simulink model "PID"  (R2023a)
settings: Solver=VariableStepAuto  StartTime=0.0  StopTime=10.0  RelTol=1e-3
settings Model: Creator=ag027  LastModifiedBy=ag027

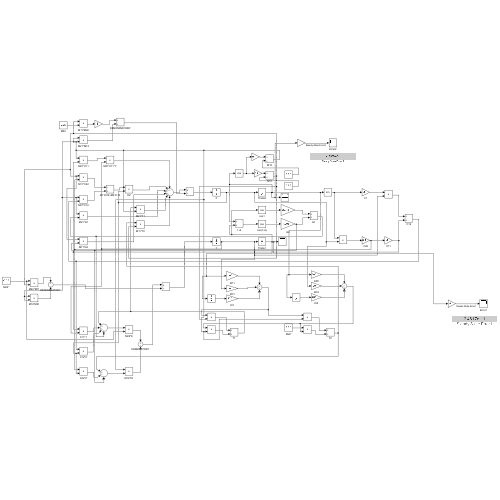
[thumbnail: Simulink's stored preview of the top-level diagram]
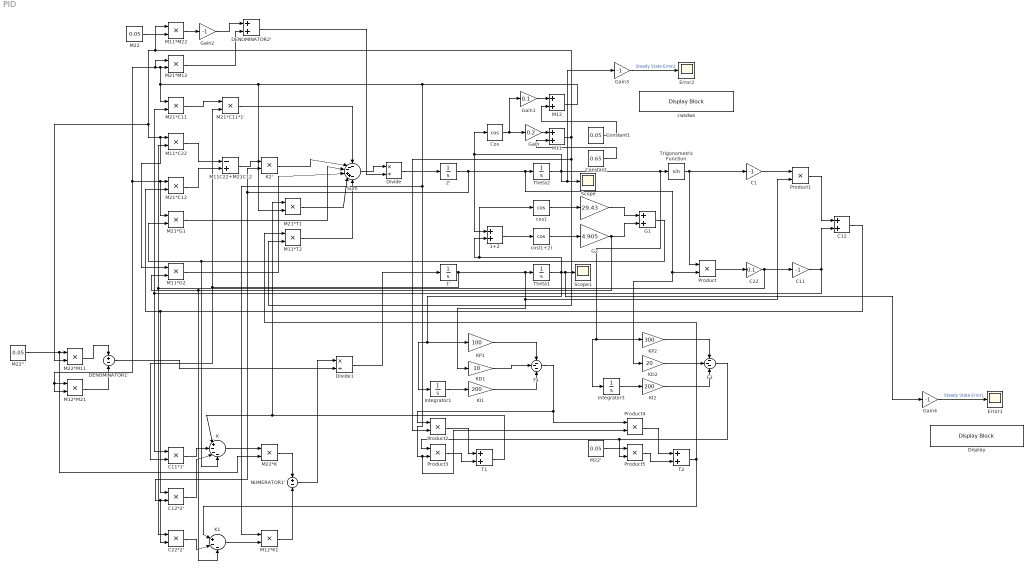
== system PID ==
  " " : Gain  Gain=29.43
  1' : Integrator
  1+2 : Sum
  2' : Integrator
  C1 : Gain  Gain=-1
  C11 : Gain  Gain=-1
  C11*1' : Product
  C12 : Sum
  C12*2' : Product
  C22 : Gain  Gain=0.1
  C22*2' : Product
  Constant : Constant  Value=0.65
  Constant1 : Constant  Value=0.05
  Cos : Trigonometry  Operator=cos
  DENOMINATOR1' : Sum  Inputs=+-
  DENOMINATOR2' : Sum
  Display : DisplayBlock  LabelPosition=Bottom  Transparency=1
  Divide : Product  Inputs=*/
  Divide1 : Product  Inputs=*/
  Error1 : Scope
  Error2 : Scope
  F1 : Sum  Inputs=---
  F2 : Sum  Inputs=---
  G1 : Sum
  G2 : Gain  Gain=4.905
  Gain : Gain  Gain=0.2
  Gain1 : Gain  Gain=0.1
  Gain2 : Gain  Gain=-1
  Gain3 : Gain  Gain=-1
  Gain4 : Gain  Gain=-1
  Integrator1 : Integrator
  Integrator3 : Integrator
  K : Sum  Inputs=|+---
  K1 : Sum  Inputs=|+--
  K2' : Product
  KD1 : Gain  Gain=10
  KD2 : Gain  Gain=20
  KI1 : Gain  Gain=200
  KI2 : Gain  Gain=200
  KP1 : Gain  Gain=100
  KP2 : Gain  Gain=300
  M11 : Sum
  M11*C22 : Product
  M11*G2 : Product
  M11*M22 : Product
  M11*T2 : Product
  M11C22+M21C12 : Sum  Inputs=-+
  M12 : Sum
  M12*K1 : Product
  M12*M21 : Product
  M21*C11 : Product
  M21*C11*1' : Product
  M21*C12 : Product
  M21*G1 : Product
  M21*M12 : Product
  M21*T1 : Product
  M22 : Constant  Value=0.05
  M22' : Constant  Value=0.05
  M22'' : Constant  Value=0.05
  M22*K : Product
  M22*M11 : Product
  NUMERATOR1' : Sum  Inputs=+-
  Product{,1..5} (6 alike) : Product
  Scope : Scope
  Scope1 : Scope
  Sum : Sum  Inputs=---++-
  T1 : Sum
  T2 : Sum
  Theta1 : Integrator  InitialCondition=0.1
  Theta2 : Integrator  InitialCondition=0.1
  Trigonometric Function : Trigonometry
  cos(1+2) : Trigonometry  Operator=cos
  cos1 : Trigonometry  Operator=cos
  cwsdws : DisplayBlock  LabelPosition=Bottom  Transparency=1
  wires:
  Constant/1 -> M11/2
  Cos/1 -> Gain1/1, Gain/1
  Gain/1 -> M11/1
  Gain1/1 -> M12/1
  Constant1/1 -> M12/2
  1'/1 -> Product1/2, KD1/1, Theta1/1, C11*1'/2, M21*C11*1'/2
  Theta1/1 -> Gain4/1, Scope1/1, cos1/1, 1+2/2, KP1/1, Integrator1/1
  1+2/1 -> cos(1+2)/1
  cos(1+2)/1 -> G2/1
  cos1/1 -> " "/1
  G2/1 -> M11*G2/2, K1/3, G1/2
  " "/1 -> G1/1
  Trigonometric Function/1 -> C1/1, Product/1
  Product/1 -> C22/1
  C22/1 -> C22*2'/1, M11*C22/2, C11/1
  C1/1 -> Product1/1
  Product1/1 -> C12/1
  C11/1 -> C12/2, C11*1'/1, M21*C11/2
  M12/1 -> Product4/2, Product3/2, M12*K1/1, M21*T1/2, M21*C11/1, M12*M21/2, M12*M21/1, M21*G1/1, M21*C12/1, M21*M12/1, M21*M12/2
  M11/1 -> M11*T2/2, Product2/2, M22*M11/2, M11*G2/1, M11*C22/1, M11*M22/1
  M22/1 -> M11*M22/2
  M11*M22/1 -> Gain2/1
  Gain2/1 -> DENOMINATOR2'/1
  M21*M12/1 -> DENOMINATOR2'/2
  M21*C11/1 -> M21*C11*1'/1
  M21*C11*1'/1 -> Sum/1
  C12/1 -> C12*2'/1, M21*C12/2
  M11*C22/1 -> M11C22+M21C12/1
  M21*C12/1 -> M11C22+M21C12/2
  M11C22+M21C12/1 -> K2'/1
  K2'/1 -> Sum/2
  G1/1 -> K/4, M21*G1/2
  M21*G1/1 -> Sum/3
  M11*G2/1 -> Sum/4
  Integrator1/1 -> KI1/1
  KP1/1 -> F1/1
  KD1/1 -> F1/2
  KI1/1 -> F1/3
  KI2/1 -> F2/3
  Integrator3/1 -> KI2/1
  2'/1 -> C22*2'/2, C12*2'/2, K2'/2, Product/2, KD2/1, Theta2/1
  KP2/1 -> F2/1
  KD2/1 -> F2/2
  F1/1 -> Product4/1, Product2/1
  F2/1 -> Product5/2, Product3/1
  Product2/1 -> T1/1
  Product3/1 -> T1/2
  Product4/1 -> T2/1
  Product5/1 -> T2/2
  M22'/1 -> Product5/1
  T1/1 -> M21*T1/1, K/1
  T2/1 -> K1/1, M11*T2/1
  M21*T1/1 -> Sum/5
  M11*T2/1 -> Sum/6
  Sum/1 -> Divide/1
  DENOMINATOR2'/1 -> Divide/2
  Divide/1 -> 2'/1
  M22''/1 -> M22*K/2, M22*M11/1
  M22*M11/1 -> DENOMINATOR1'/1
  M12*M21/1 -> DENOMINATOR1'/2
  C11*1'/1 -> K/2
  C12*2'/1 -> K/3
  K/1 -> M22*K/1
  C22*2'/1 -> K1/2
  K1/1 -> M12*K1/2
  M22*K/1 -> NUMERATOR1'/1
  M12*K1/1 -> NUMERATOR1'/2
  NUMERATOR1'/1 -> Divide1/1
  DENOMINATOR1'/1 -> Divide1/2
  Divide1/1 -> 1'/1
  Theta2/1 -> Gain3/1, Scope/1, KP2/1, Integrator3/1, Trigonometric Function/1, 1+2/1, Cos/1
  Gain3/1 -> Error2/1  "Steady State Error2"
  Gain4/1 -> Error1/1  "Steady State Error1"
